simulink model "task_1"  (Simulink 7.6)
settings: Solver=ode45  StartTime=1.0  StopTime=2.0  RelTol=1e-3
settings Model: Creator=Admin  LastModifiedBy=Admin

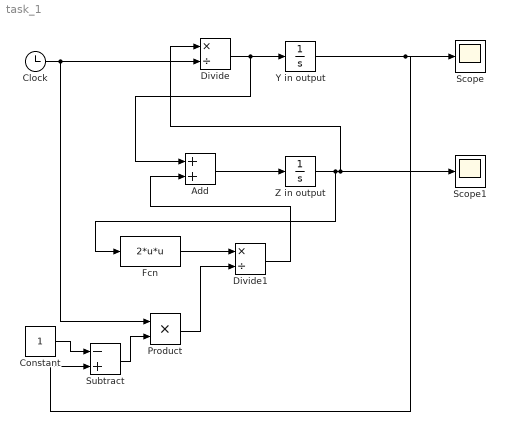
== system task_1 ==
  Add : Sum
  Clock : Clock
      settings: Decimation=10
  Constant : Constant
  Divide : Product  Inputs=*/
  Divide1 : Product  Inputs=*/
  Fcn : Fcn  Expr=2*u*u
  Product : Product  RndMeth=Zero
  Scope : Scope
      settings: Tag=Y func
  Scope1 : Scope
  Subtract : Sum  Inputs=-+
  Y in output : Integrator
  Z in output : Integrator  InitialCondition=1/3
  wires:
  Divide/1 -> Y in output/1, Add/1
  Clock/1 -> Divide/2, Product/1
  Z in output/1 -> Fcn/1, Divide/1, Scope1/1
  Add/1 -> Z in output/1
  Fcn/1 -> Divide1/1
  Product/1 -> Divide1/2
  Subtract/1 -> Product/2
  Y in output/1 -> Subtract/2, Scope/1
  Constant/1 -> Subtract/1
  Divide1/1 -> Add/2
